simulink model "diagrama_sugeno"  (Simulink 7.9)
settings: Solver=ode3  StartTime=0.0  StopTime=200  FixedStep=0.1  RelTol=1e-3
libraries: fuzblock x1
settings Model: Creator=DanielFrutuoso  LastModifiedBy=DanielFrutuoso
settings SolverCC: ZeroCrossControl=DisableAll

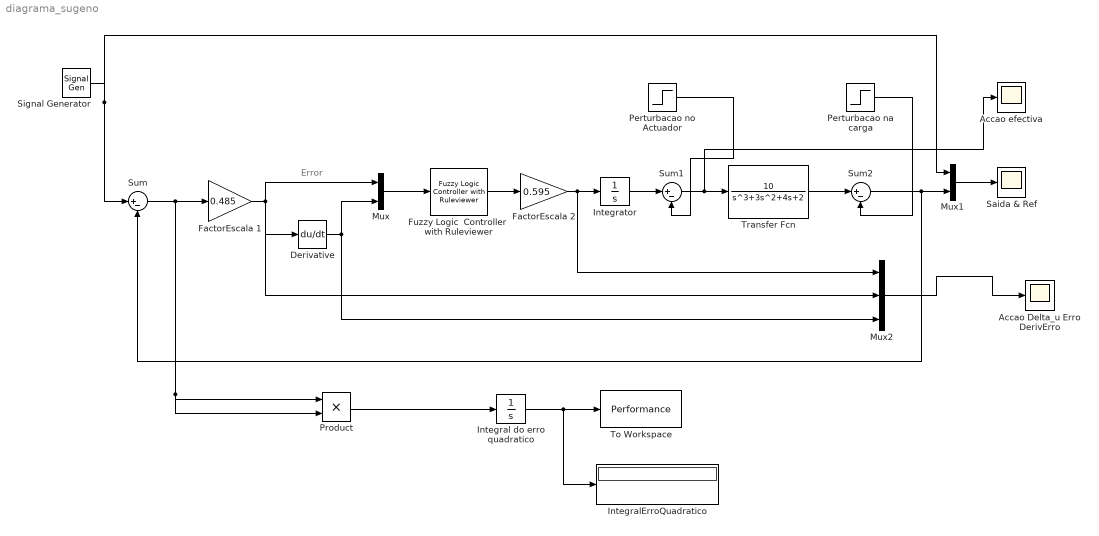
== system diagrama_sugeno ==
  note: Error
  Accao Delta_u Erro DerivErro : Scope
      settings: YMin=-0.1  YMax=0.07  SaveName=ScopeData3
  Accao efectiva : Scope
  Derivative : Derivative
  FactorEscala 1 : Gain  Gain=0.485
  FactorEscala 2 : Gain  Gain=0.595
  Fuzzy Logic  Controller  with Ruleviewer : fuzblock/Fuzzy Logic  Controller  with Ruleviewer  fismatrix=fis_sugeno  Ts=0.5
  Integral do erro quadratico : Integrator
  IntegralErroQuadratico : Display
      settings: Decimation=2
  Integrator : Integrator
  Mux : Mux  Inputs=2
  Mux1 : Mux  Inputs=2
  Mux2 : Mux  Inputs=3
  Perturbacao na carga : Step  Time=120  After=-1  SampleTime=0
  Perturbacao no Actuador : Step  Time=50  After=-1  SampleTime=0
  Product : Product  RndMeth=Zero
  Saida & Ref : Scope
      settings: YMin=-1.25  YMax=3.75
  Signal Generator : SignalGenerator  Frequency=0.025
  Sum : Sum  Inputs=|+-
  Sum1 : Sum  Inputs=|+-
  Sum2 : Sum  Inputs=|+-
  To Workspace : ToWorkspace  VariableName=Performance  SampleTime=-1  SaveFormat=Timeseries
  Transfer Fcn : TransferFcn  Numerator=[10]  Denominator=[1 3 4 2]
  wires:
  Signal Generator/1 -> Mux1/1, Sum/1
  Sum/1 -> Product/1, Product/2, FactorEscala 1/1
  FactorEscala 1/1 -> Mux2/2, Mux/1, Derivative/1
  Derivative/1 -> Mux/2, Mux2/3
  Mux/1 -> Fuzzy Logic  Controller  with Ruleviewer/1
  Fuzzy Logic  Controller  with Ruleviewer/1 -> FactorEscala 2/1
  FactorEscala 2/1 -> Integrator/1, Mux2/1
  Integrator/1 -> Sum1/1
  Sum1/1 -> Transfer Fcn/1, Accao efectiva/1
  Transfer Fcn/1 -> Sum2/1
  Perturbacao no Actuador/1 -> Sum1/2
  Perturbacao na carga/1 -> Sum2/2
  Sum2/1 -> Mux1/2, Sum/2
  Mux1/1 -> Saida & Ref/1
  Integral do erro quadratico/1 -> To Workspace/1, IntegralErroQuadratico/1
  Product/1 -> Integral do erro quadratico/1
  Mux2/1 -> Accao Delta_u Erro DerivErro/1
